simulink model "ADRC"  (R2020b)
settings: Solver=VariableStepAuto  StartTime=0.0  StopTime=10.0  RelTol=1e-3
settings Model: Creator=jswl  LastModifiedBy=jswl

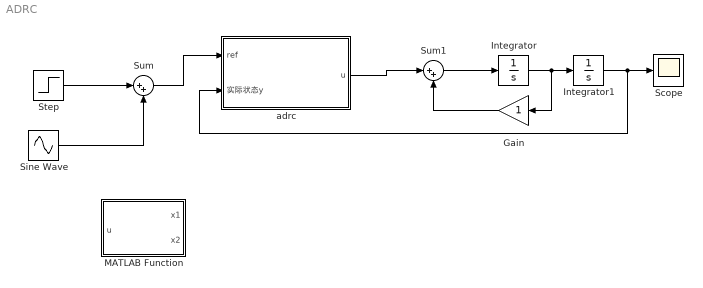
== system ADRC ==
  Gain : Gain
  Integrator : Integrator
  Integrator1 : Integrator
  MATLAB Function : MATLAB Function  TreatAsAtomicUnit=on
  Scope : Scope
  Sine Wave : Sin  SampleTime=0
  Step : Step  SampleTime=0
  Sum : Sum  Inputs=|++
  Sum1 : Sum  Inputs=|++
  adrc : Subsystem  mask{Wc=2, W0=10, b0=1}
  wires:
  Step/1 -> Sum/1
  Sine Wave/1 -> Sum/2
  Sum/1 -> adrc/1(ref)
  adrc/1(u) -> Sum1/1
  Sum1/1 -> Integrator/1
  Integrator/1 -> Gain/1, Integrator1/1
  Integrator1/1 -> Scope/1, adrc/2(实际状态y)
  Gain/1 -> Sum1/2

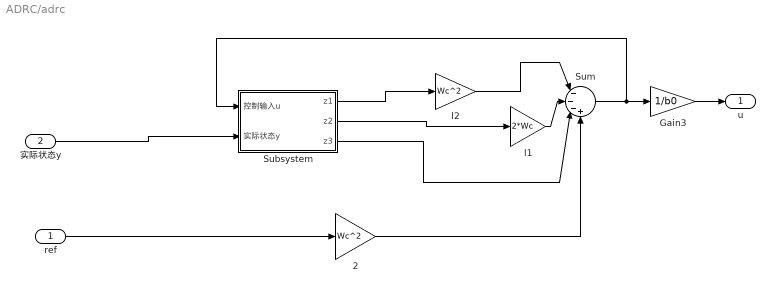
== system ADRC/adrc ==
  ref : Inport
  实际状态y : Inport  Port=2
  2 : Gain  Gain=Wc^2
  Gain3 : Gain  Gain=1/b0
  Subsystem : Subsystem
  Sum : Sum  Inputs=|---+
  l1 : Gain  Gain=2*Wc
  l2 : Gain  Gain=Wc^2
  u : Outport  VectorParamsAs1DForOutWhenUnconnected=off
  wires:
  实际状态y/1 -> Subsystem/2(实际状态y)
  Sum/1 -> Subsystem/1(控制输入u), Gain3/1
  2/1 -> Sum/4
  l2/1 -> Sum/1
  Subsystem/3(z3) -> Sum/3
  l1/1 -> Sum/2
  Subsystem/2(z2) -> l1/1
  Subsystem/1(z1) -> l2/1
  ref/1 -> 2/1
  Gain3/1 -> u/1

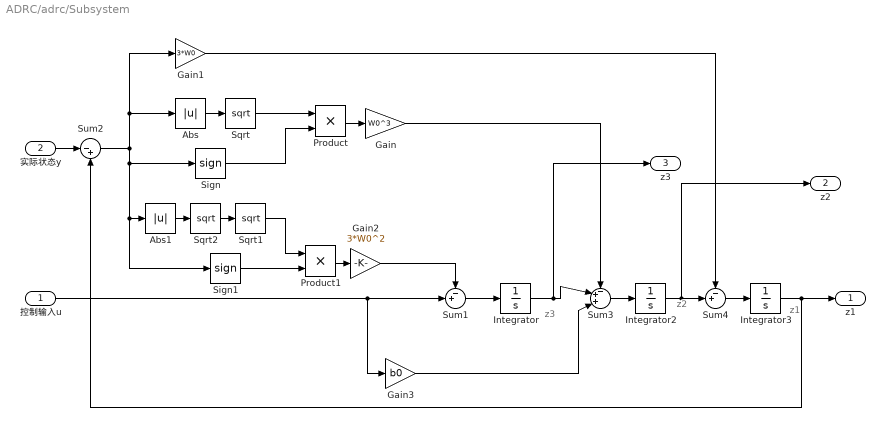
== system ADRC/adrc/Subsystem ==
  note: z1
  note: z2
  note: z3
  控制输入u : Inport
  实际状态y : Inport  Port=2
  Abs : Abs
  Abs1 : Abs
  Gain : Gain  Gain=W0^3
  Gain1 : Gain  Gain=3*W0
  Gain2 : Gain  Gain=3*W0^2
  Gain3 : Gain  Gain=b0
  Integrator : Integrator
  Integrator2 : Integrator
  Integrator3 : Integrator
  Product : Product
  Product1 : Product
  Sign : Signum
  Sign1 : Signum
  Sqrt : Sqrt  SaturateOnIntegerOverflow=on
  Sqrt1 : Sqrt  SaturateOnIntegerOverflow=on
  Sqrt2 : Sqrt  SaturateOnIntegerOverflow=on
  Sum1 : Sum  Inputs=-+|
  Sum2 : Sum  Inputs=|-+
  Sum3 : Sum  Inputs=-++|
  Sum4 : Sum  Inputs=-+|
  z1 : Outport  VectorParamsAs1DForOutWhenUnconnected=off
  z2 : Outport  Port=2
  z3 : Outport  Port=3
  wires:
  Sum2/1 -> Abs/1, Gain1/1, Sign1/1, Abs1/1, Sign/1
  Sign1/1 -> Product1/2
  Integrator2/1 -> z2/1, Sum4/2
  Sum4/1 -> Integrator3/1
  Integrator3/1 -> z1/1, Sum2/2
  Abs1/1 -> Sqrt2/1
  Product/1 -> Gain/1
  实际状态y/1 -> Sum2/1
  Abs/1 -> Sqrt/1
  Integrator/1 -> z3/1, Sum3/2
  Sqrt1/1 -> Product1/1
  Sqrt/1 -> Product/1
  Sum3/1 -> Integrator2/1
  Sqrt2/1 -> Sqrt1/1
  Gain/1 -> Sum3/1
  Sum1/1 -> Integrator/1
  Gain1/1 -> Sum4/1
  Gain2/1 -> Sum1/1
  控制输入u/1 -> Gain3/1, Sum1/2
  Product1/1 -> Gain2/1
  Gain3/1 -> Sum3/3
  Sign/1 -> Product/2

== matlab function ADRC/MATLAB Function ==
  data: u input; x1 output; x2 output
function [x1,x2] = TD_2order(u)
T=0.001;
r=100;
h=0.001;
persistent x_1 x_2
if isempty(x_1)
    x_1=u;
    x_2=0;
end
x1k=x_1;
x2k=x_2;
x_1=x1k+T*x2k;
x_2=x2k+T*fst(x1k,x2k,u,r,h);
x1=x_1;
x2=x_2;
end

function f=fst(x1,x2,u,r,h)
d=r*h;			%h为滤波因子  r为调节系数，r越大跟踪效果越好，但微分信号会增加高频噪声
d0=d*h;	%反之，微分信号越平滑，会产生一定的滞后
y=x1-u+h*x2;
a0=sqrt(d^2+8*r*abs(y));
if abs(y)<=d0
    a=x2+y/h;
else
    a=x2+0.5*(a0-d)*sign(y);
end
if abs(a)<=d
    f=-r*a/d;
else
    f=-r*sign(a);
end
end
